simulink model "scw_ut"  (Simulink 8.1)
settings: Solver=FixedStepDiscrete  StartTime=0.0  StopTime=10.0  FixedStep=5e-3  RelTol=1e-3
undefined symbols (not defined in the file or in its folder): KFCW_BrakePreFillTimer_ms, KFCW_HapticOnTimer_ms
libraries: siltestlib x16, scw x1
settings Model: Creator=xsellart  LastModifiedBy=AT015411
settings DataIOCC: SignalLoggingSaveFormat=Dataset
settings OptimizationCC: ExpressionDepthLimit=128
settings DebuggingCC: FcnCallInpInsideContextMsg=EnableAllAsError
settings GRTTargetCC: CombineOutputUpdateFcns=on  GRTInterface=off

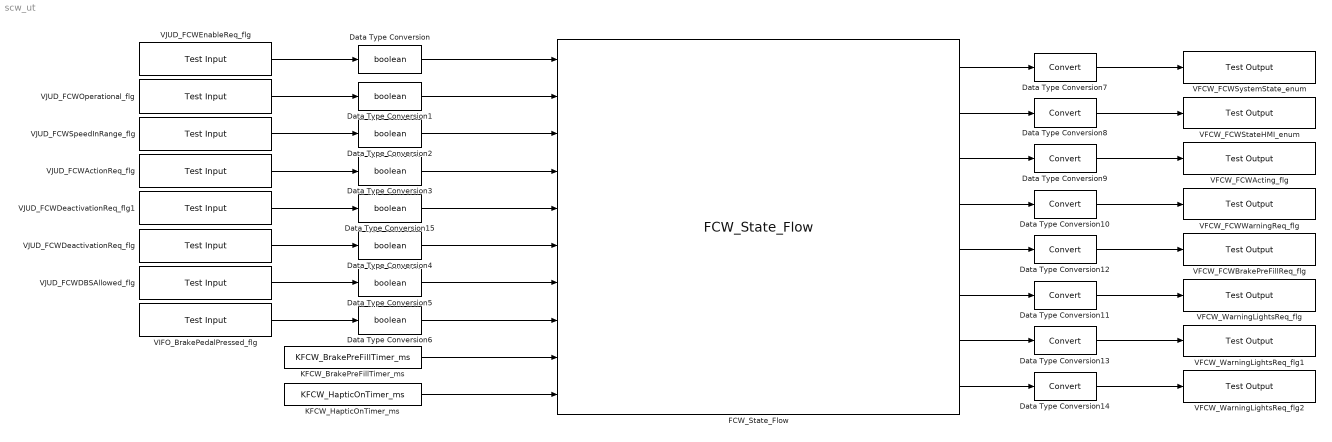
== system scw_ut ==
  Data Type Conversion{,1..6,15} (8 alike) : DataTypeConversion  OutDataTypeStr=boolean
  Data Type Conversion{7..14} (8 alike) : DataTypeConversion
  FCW_State_Flow : scw/FCW_State_Flow
  KFCW_BrakePreFillTimer_ms : Constant  Value=KFCW_BrakePreFillTimer_ms
  KFCW_HapticOnTimer_ms : Constant  Value=KFCW_HapticOnTimer_ms
  VFCW_FCWActing_flg : siltestlib/Test Output  varname=VFCW_FCWActing_flg  sampletime=-1
  VFCW_FCWBrakePreFillReq_flg : siltestlib/Test Output  varname=VFCW_FCWBrakePreFillReq_flg  sampletime=-1
  VFCW_FCWStateHMI_enum : siltestlib/Test Output  varname=VFCW_FCWStateHMI_enum  sampletime=-1
  VFCW_FCWSystemState_enum : siltestlib/Test Output  varname=VFCW_FCWSystemState_enum  sampletime=-1
  VFCW_FCWWarningReq_flg : siltestlib/Test Output  varname=VFCW_FCWWarningReq_flg  sampletime=-1
  VFCW_WarningLightsReq_flg : siltestlib/Test Output  varname=VFCW_FCWBrakePreFillReqAppl_flg  sampletime=-1
  VFCW_WarningLightsReq_flg1 : siltestlib/Test Output  varname=VFCW_FCWHapticReq_flg  sampletime=-1
  VFCW_WarningLightsReq_flg2 : siltestlib/Test Output  varname=VFCW_FCWDecelReqAppl_flg  sampletime=-1
  VIFO_BrakePedalPressed_flg : siltestlib/Test Input  varname=VIFO_BrakePedalPressed_flg  sampletime=-1
  VJUD_FCWActionReq_flg : siltestlib/Test Input  varname=VJUD_FCWActionReq_flg  sampletime=-1
  VJUD_FCWDBSAllowed_flg : siltestlib/Test Input  varname=VJUD_FCWDBSAllowed_flg  sampletime=-1
  VJUD_FCWDeactivationReq_flg : siltestlib/Test Input  varname=VJUD_FCWDeactivationReq_flg  sampletime=-1
  VJUD_FCWDeactivationReq_flg1 : siltestlib/Test Input  varname=VJUD_FCWReturnOperational_flg  sampletime=-1
  VJUD_FCWEnableReq_flg : siltestlib/Test Input  varname=VJUD_FCWEnableReq_flg  sampletime=-1
  VJUD_FCWOperational_flg : siltestlib/Test Input  varname=VJUD_FCWOperational_flg  sampletime=-1
  VJUD_FCWSpeedInRange_flg : siltestlib/Test Input  varname=VJUD_FCWSpeedInRange_flg  sampletime=-1
  wires:
  VJUD_FCWEnableReq_flg/1 -> Data Type Conversion/1
  VJUD_FCWOperational_flg/1 -> Data Type Conversion1/1
  VJUD_FCWSpeedInRange_flg/1 -> Data Type Conversion2/1
  VJUD_FCWActionReq_flg/1 -> Data Type Conversion3/1
  VJUD_FCWDeactivationReq_flg/1 -> Data Type Conversion4/1
  VJUD_FCWDBSAllowed_flg/1 -> Data Type Conversion5/1
  VIFO_BrakePedalPressed_flg/1 -> Data Type Conversion6/1
  Data Type Conversion1/1 -> FCW_State_Flow/2
  Data Type Conversion/1 -> FCW_State_Flow/1
  Data Type Conversion11/1 -> VFCW_WarningLightsReq_flg/1
  FCW_State_Flow/1 -> Data Type Conversion7/1
  FCW_State_Flow/2 -> Data Type Conversion8/1
  FCW_State_Flow/3 -> Data Type Conversion9/1
  FCW_State_Flow/4 -> Data Type Conversion10/1
  FCW_State_Flow/5 -> Data Type Conversion12/1
  Data Type Conversion7/1 -> VFCW_FCWSystemState_enum/1
  Data Type Conversion8/1 -> VFCW_FCWStateHMI_enum/1
  Data Type Conversion9/1 -> VFCW_FCWActing_flg/1
  Data Type Conversion10/1 -> VFCW_FCWWarningReq_flg/1
  Data Type Conversion12/1 -> VFCW_FCWBrakePreFillReq_flg/1
  Data Type Conversion2/1 -> FCW_State_Flow/3
  Data Type Conversion3/1 -> FCW_State_Flow/4
  Data Type Conversion4/1 -> FCW_State_Flow/6
  Data Type Conversion6/1 -> FCW_State_Flow/8
  FCW_State_Flow/6 -> Data Type Conversion11/1
  Data Type Conversion13/1 -> VFCW_WarningLightsReq_flg1/1
  FCW_State_Flow/7 -> Data Type Conversion13/1
  Data Type Conversion14/1 -> VFCW_WarningLightsReq_flg2/1
  FCW_State_Flow/8 -> Data Type Conversion14/1
  Data Type Conversion5/1 -> FCW_State_Flow/7
  VJUD_FCWDeactivationReq_flg1/1 -> Data Type Conversion15/1
  Data Type Conversion15/1 -> FCW_State_Flow/5
  KFCW_BrakePreFillTimer_ms/1 -> FCW_State_Flow/9
  KFCW_HapticOnTimer_ms/1 -> FCW_State_Flow/10
